simulink model "top"  (R2015a)
settings: Solver=ode3  StartTime=0.0  StopTime=10  RelTol=1e-3
settings Model: SimulationMode=rapid-accelerator  Creator=andersor  LastModifiedBy=ktadepal
settings SolverCC: AutoInsertRateTranBlk=on
settings DataIOCC: LimitDataPoints=off  SaveFormat=StructureWithTime  DSMLogging=off  SaveTime=off  ReturnWorkspaceOutputs=on
settings OptimizationCC: InlineParams=on  UseDivisionForNetSlopeComputation=UseDivisionForReciprocalsOfIntegersOnly  EnhancedBackFolding=on  ExpressionDepthLimit=2147483647  EfficientMapNaN2IntZero=off  LifeSpan=1
settings DebuggingCC: ConsistencyChecking=warning  SignalRangeChecking=error  ReadBeforeWriteMsg=DisableAll  WriteAfterWriteMsg=DisableAll  WriteAfterReadMsg=DisableAll  AlgebraicLoopMsg=none  ArtificialAlgebraicLoopMsg=none  CheckSSInitialOutputMsg=off  MaxConsecutiveZCsMsg=warning  InheritedTsInSrcMsg=none  DiscreteInheritContinuousMsg=none  MultiTaskDSMMsg=none  MultiTaskRateTransMsg=warning  TasksWithSamePriorityMsg=none  SigSpecEnsureSampleTimeMsg=none  CheckMatrixSingularityMsg=error  IntegerOverflowMsg=none  ParameterDowncastMsg=none  ParameterOverflowMsg=none  ParameterPrecisionLossMsg=none  ParameterTunabilityLossMsg=none  UnconnectedInputMsg=none  UnconnectedOutputMsg=none  UnconnectedLineMsg=none  ModelReferenceIOMsg=warning  ModelReferenceIOMismatchMessage=warning  UnknownTsInhSupMsg=none  SimStateInterfaceChecksumMismatchMsg=none  StrictBusMsg=ErrorOnBusTreatedAsVector  BusNameAdapt=ErrorWithoutRepair  SFInvalidInputDataAccessInChartInitDiag=error  SFNoUnconditionalDefaultTransitionDiag=error  IntegerSaturationMsg=none
settings HardwareCC: ProdBitPerLong=64  ProdBitPerPointer=64  ProdIntDivRoundTo=Zero  ProdEndianess=LittleEndian  ProdWordSize=64  ProdHWDeviceType=Intel->x86-64  TargetLongLongMode=on  TargetIntDivRoundTo=Zero  TargetEndianess=LittleEndian  TargetHWDeviceType=Generic->MATLAB Host Computer
settings ModelReferenceCC: UpdateModelReferenceTargets=Force  ParallelModelReferenceMATLABWorkerInit=Load Top Model  PropagateVarSize=Only when enabling  ModelReferencePassRootInputsByReference=off  PropagateSignalLabelsOutOfModel=on
settings RTWCC: SystemTargetFile=ert.tlc  TemplateMakefile=ert_default_tmf  Description=Embedded Coder  GenerateReport=on  IncludeHyperlinkInReport=on  LaunchReport=on  GenerateTraceInfo=on  GenerateTraceReport=on  GenerateTraceReportSl=on  GenerateTraceReportSf=on  GenerateTraceReportEml=on
settings CodeAppCC: ForceParamTrailComments=on  IgnoreCustomStorageClasses=off  SimulinkDataObjDesc=on  SFDataObjDesc=on  MangleLength=14  CustomSymbolStrGlobalVar=$N$M  CustomSymbolStrType=$N$M  CustomSymbolStrField=$M$N_$A  CustomSymbolStrFcn=$M$N  CustomSymbolStrFcnArg=_$Nr1_666$M$I  CustomSymbolStrBlkIO=$N$M$ART15  CustomSymbolStrTmpVar=$N$M$R  CustomSymbolStrMacro=$N$M  InsertBlockDesc=on  ReqsInCode=on
settings ERTTargetCC: CodeReplacementLibrary=GNU99 (GNU)  ParMdlRefBuildCompliant=on  CompOptLevelCompliant=on  ConcurrentExecutionCompliant=on  IncludeMdlTerminateFcn=off  GeneratePreprocessorConditionals=Disable all  CombineSignalStateStructs=on  ERTFirstTimeCompliant=on  IncludeFileDelimiter=UseBracket  LogVarNameModifier=none  MatFileLogging=on  SupportContinuousTime=off  SupportNonInlinedSFcns=on  ParenthesesLevel=Minimum  ModelStepFunctionPrototypeControlCompliant=on  CPPClassGenCompliant=on  InlinedParameterPlacement=Hierarchical  MultiInstanceErrorCode=Warning  ERTCustomFileTemplate=example_file_process.tlc  EnableDataOwnership=on  SignalDisplayLevel=2  ParamTuneLevel=7  GlobalDataDefinition=InSourceFile  DataDefinitionFile=global2.c  DataReferenceFile=global2.h  ConvertIfToSwitch=on  IndentStyle=Allman  IndentSize=7  MinIdInt32=IAT_MIN_int32  MaxIdUint8=IAT_MAX_uint8

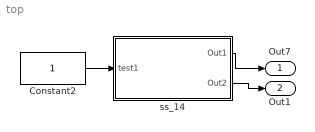
== system top ==
  Constant2 : Constant
  ss_14 : Subsystem  TreatAsAtomicUnit=on
      settings: MinAlgLoopOccurrences=on  RTWFileNameOpts=Use subsystem name
  Out7 : Outport
  Out1 : Outport  Port=2
  wires:
  ss_14/1(Out1) -> Out7/1
  Constant2/1 -> ss_14/1(test1)
  ss_14/2(Out2) -> Out1/1

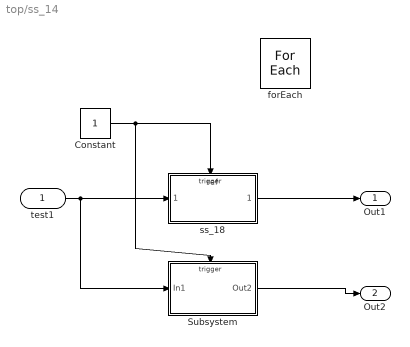
== system top/ss_14 ==
  test1 : Inport  Partition=on  PartitionDimension=1  PartitionWidth=1
  Constant : Constant  OutDataTypeStr=boolean  SampleTime=-1
  Subsystem : Subsystem
  forEach : ForEach
  ss_18 : ModelReference  ModelNameDialog=ref.slx  ModelReferenceVersion=1.259  CopyOfModelName=ref.slx  TriggerPortName=Trigger  TriggerPortTriggerType=rising
  Out1 : Outport  ConcatenationDimension=1
  Out2 : Outport  Port=2  ConcatenationDimension=1
  wires:
  ss_18/1 -> Out1/1
  Constant/1 -> ss_18/Trigger, Subsystem/Trigger
  test1/1 -> Subsystem/1(In1), ss_18/1
  Subsystem/1(Out2) -> Out2/1

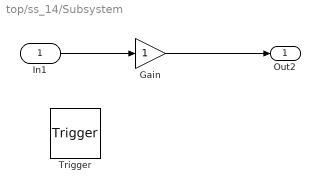
== system top/ss_14/Subsystem ==
  In1 : Inport  OutDataTypeStr=double  PortDimensions=1  Interpolate=off
  Trigger : TriggerPort  StatesWhenEnabling=reset  PropagateVarSize=Only when enabling  ShowOutputPort=on  OutputDataType=double  SampleTime=-1  PortDimensions=1  TriggerSignalSampleTime=[0.10000000000000001,0]  OutDataTypeStr=boolean
  Gain : Gain
  Out2 : Outport  InitialOutput=4
  wires:
  In1/1 -> Gain/1
  Gain/1 -> Out2/1
